simulink model "MKIV_build_simulink_flight_outer20210320_no1"  (R2016b)
settings: Solver=FixedStepDiscrete  StartTime=0.0  StopTime=inf  RelTol=1e-3
PostLoadFcn:
  | kFactor = 1.2;
  | 
  | KpRollAttitude = 0.630138625117681 / kFactor;
  | KiRollAttitude = 0.0552303199591522 / kFactor;
  | 
  | KpPitchAttitude = 0.630138625117681 / kFactor;
  | KiPitchAttitude = 0.0552303199591522 / kFactor;
  | 
  | KpRollRate = 1.31533836563383 / kFactor;
  | KiRollRate = 0.460338699849681 / kFactor;
  | 
  | KpPitchRate = 1.31533836563383 / kFactor;
  | KiPitchRate = 0.460338699849681 / kFactor;
  | 
  | KpYawRate = 1.31533836563383 / kFactor;
  | KiYawRate = 0.460338699849681 / kFactor;
undefined symbols (not defined in the file): PX4_TUNE_ENUM, RGBLED_COLOR_ENUM, RGBLED_MODE_ENUM
libraries: pixhawk_slib_sensors_actuators x8, pixhawk_slib_ADC_serial x1, pixhawk_slib_uORB_RW x1, pixhawk_slib_misc_utils x1
settings Model: Creator=Steve  LastModifiedBy=scott
settings SolverCC: AutoInsertRateTranBlk=on
settings DataIOCC: LimitDataPoints=on  SaveFormat=Array
settings OptimizationCC: DefaultParameterBehavior=Inlined  LifeSpan=1  MaxStackSize=64
settings DebuggingCC: SolverPrmCheckMsg=warning  AllowSymbolicDim=off  SFUnexpectedBacktrackingDiag=warning  SFNoUnconditionalDefaultTransitionDiag=warning  SFExecutionAtInitializationDiag=none
settings HardwareCC: ProdBitPerPointer=32  ProdBitPerSizeT=32  ProdBitPerPtrDiffT=32  ProdLargestAtomicInteger=Long  ProdLargestAtomicFloat=Double  ProdWordSize=32  ProdHWDeviceType=ARM Compatible->ARM Cortex
settings ModelReferenceCC: PropagateSignalLabelsOutOfModel=off
settings RTWCC: SystemTargetFile=ert.tlc  HardwareBoard=Pixhawk PX4  TemplateMakefile=ert_default_tmf  Description=Embedded Coder  GenerateReport=on  Toolchain=Pixhawk Toolchain  IncludeHyperlinkInReport=on  LaunchReport=on  GenerateTraceReport=on  GenerateTraceReportSl=on  GenerateTraceReportSf=on  GenerateTraceReportEml=on  GenerateCodeMetricsReport=on
settings CodeAppCC: IgnoreCustomStorageClasses=off
settings ERTTargetCC: CodeReplacementLibrary=GCC ARM Cortex-A9  ExtModeTransport=1  ExtModeMexFile=ext_serial_win32_comm  ExtModeMexArgs=/dev/serial  ERTCustomFileTemplate=PX4_codertarget_file_process.tlc  ConvertIfToSwitch=off  SuppressUnreachableDefaultCases=off
settings ConfigComp: CovMetricSettings=dw  CovHtmlReporting=on  CovSaveCumulativeToWorkspaceVar=on  CovSaveSingleToWorkspaceVar=on  CovExternalEMLEnable=off  CovSFcnEnable=off

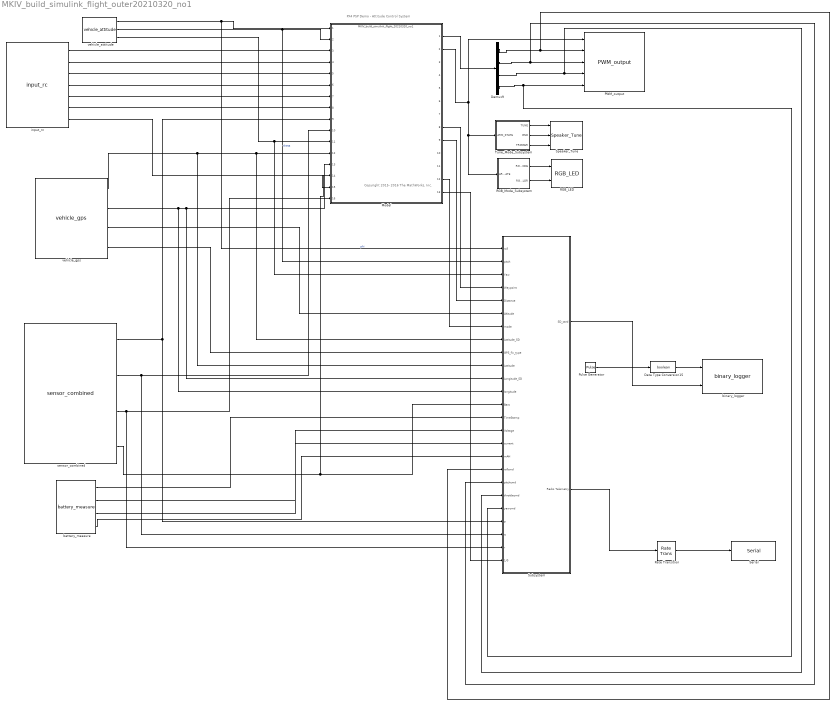
== system MKIV_build_simulink_flight_outer20210320_no1 ==
  note: PX4 PSP Demo - Attitude Control System
  note: Copyright 2015- 2016 The MathWorks, Inc.
  Data Type Conversion15 : DataTypeConversion  OutDataTypeStr=boolean
  Demux9 : Demux
  Model : ModelReference  ModelNameDialog=MKIV_build_simulink_flight_20210320_no1.slx  SimulationMode=Normal  ModelReferenceVersion=1.475
  PWM_output : pixhawk_slib_sensors_actuators/PWM_output  pwm_rate=50Hz  show_pwm1=on  show_pwm2=on  show_pwm3=on  show_pwm4=on  show_pwm5=off  show_pwm6=off  show_pwm7=off  show_pwm8=off
  Pulse Generator : DiscretePulseGenerator  Period=10  PulseWidth=5  SampleTime=10
  RGB_LED : pixhawk_slib_sensors_actuators/RGB_LED
  RGB_Mode_Subsystem : Subsystem
  Rate Transition : RateTransition  OutPortSampleTime=0.3
  Serial : pixhawk_slib_ADC_serial/Serial  DeviceName=/dev/ttyS1  ReadOrWrite=Writing  BaudRateStr=57600  block=on  WriteStatus=on  Terminator=off  Header=off  NumBytesRead=4  TerminatorChar=\n  HeaderData=57600  SimulateUsing=Code generation
  Speaker_Tune : pixhawk_slib_sensors_actuators/Speaker_Tune
  Subsystem : Subsystem
  Tune_Mode_Subsystem : Subsystem
  battery_measure : pixhawk_slib_sensors_actuators/battery_measure  SampleTime=1/250  VoltageOut=on  VoltageFilteredOut=off  CurrentOut=on  mAH_Out=on  TimeStamp=on
  binary_logger : pixhawk_slib_misc_utils/binary_logger  logfile=/fs/microsd/log  cacheflag=off  numRecs=1000
  input_rc : pixhawk_slib_sensors_actuators/input_rc  sampletime=1/250  channel1=on  channel2=on  channel3=on  channel4=on  channel5=on  channel6=on  channel7=on  channel8=off  ch_count=off  rssi=off  rc_failsafe=off  rc_lost=off  rc_inputsource=off
  sensor_combined : pixhawk_slib_sensors_actuators/sensor_combined  sampletime=1/250  show_mag=off  show_acc=off  show_gyro=on  show_baro=on  show_ts=off
  vehicle_attitude : pixhawk_slib_sensors_actuators/vehicle_attitude  sampletime=1/250  show_r=on  show_p=on  show_y=on  show_q=off
  vehicle_gps : pixhawk_slib_sensors_actuators/vehicle_gps  sampletime=1/250  show_ts_pos=off  show_alt=on  show_ts_gps=off  show_vel=off  show_fixtype=on  show_numsat=off
  wires:
  RGB_Mode_Subsystem/1(RGB_MODE) -> RGB_LED/1
  RGB_Mode_Subsystem/2(RGB_COLOR) -> RGB_LED/2
  Tune_Mode_Subsystem/1(TUNE) -> Speaker_Tune/1
  Tune_Mode_Subsystem/2(GND) -> Speaker_Tune/2
  Tune_Mode_Subsystem/3(TRIGGER) -> Speaker_Tune/3
  Model/2 -> RGB_Mode_Subsystem/1(ARM_STATE), Tune_Mode_Subsystem/1(ARM_STATE), PWM_output/1
  vehicle_attitude/2 -> Model/2, Subsystem/2(pitch)  "theta"
  input_rc/1 -> Model/3
  input_rc/2 -> Model/4
  input_rc/3 -> Model/5
  input_rc/4 -> Model/6
  input_rc/5 -> Model/7
  Model/1 -> Demux9/1
  input_rc/6 -> Model/8
  Rate Transition/1 -> Serial/1
  Subsystem/2(Radio Telemetry) -> Rate Transition/1
  vehicle_gps/1 -> Subsystem/8(Latitude_SD), Model/12, Subsystem/10(Latitude)
  vehicle_gps/2 -> Model/13, Subsystem/11(Longitude_SD), Subsystem/12(Iongitude)
  Data Type Conversion15/1 -> binary_logger/1
  Pulse Generator/1 -> Data Type Conversion15/1
  sensor_combined/4 -> Subsystem/13(Baro), Model/14
  input_rc/7 -> Model/15
  Model/8 -> Subsystem/4(Waypoint)
  Model/9 -> Subsystem/5(Distance)
  vehicle_gps/3 -> Subsystem/6(Altitude)
  Model/12 -> Subsystem/7(mode)
  vehicle_gps/4 -> Subsystem/9(GPS_fix_type)
  battery_measure/1 -> Subsystem/14(TimeStamp)
  battery_measure/2 -> Subsystem/15(Voltage)
  battery_measure/3 -> Subsystem/16("current ")
  battery_measure/4 -> Subsystem/17(mAH)
  Subsystem/1(SD_card) -> binary_logger/2
  Demux9/1 -> Subsystem/18(rollcmd), PWM_output/2
  Demux9/2 -> Subsystem/19(pitchcmd), PWM_output/3
  Demux9/3 -> Subsystem/20(throttlecmd), PWM_output/4
  Demux9/4 -> Subsystem/21(yawcmd), PWM_output/5
  sensor_combined/1 -> Model/9, Subsystem/22(p)
  sensor_combined/2 -> Subsystem/23(q), Model/10
  sensor_combined/3 -> Model/16, Subsystem/24(r)
  Model/13 -> Subsystem/25(1/0)
  vehicle_attitude/1 -> Subsystem/1(roll), Model/1  "phi"
  vehicle_attitude/3 -> Subsystem/3(Yaw), Model/11

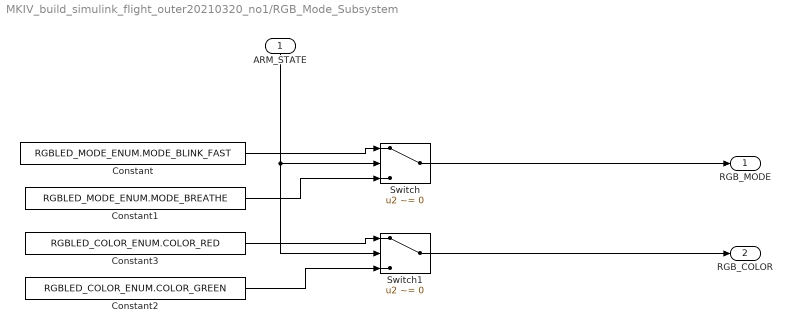
== system MKIV_build_simulink_flight_outer20210320_no1/RGB_Mode_Subsystem ==
  ARM_STATE : Inport
  Constant : Constant  Value=RGBLED_MODE_ENUM.MODE_BLINK_FAST  OutDataTypeStr=Enum: RGBLED_MODE_ENUM
  Constant1 : Constant  Value=RGBLED_MODE_ENUM.MODE_BREATHE  OutDataTypeStr=Enum: RGBLED_MODE_ENUM
  Constant2 : Constant  Value=RGBLED_COLOR_ENUM.COLOR_GREEN  OutDataTypeStr=Enum: RGBLED_COLOR_ENUM
  Constant3 : Constant  Value=RGBLED_COLOR_ENUM.COLOR_RED  OutDataTypeStr=Enum: RGBLED_COLOR_ENUM
  Switch : Switch  Criteria=u2 ~= 0  Threshold=1500  SampleTime=1/2
  Switch1 : Switch  Criteria=u2 ~= 0  Threshold=1500  SampleTime=1/2
  RGB_MODE : Outport
  RGB_COLOR : Outport  Port=2
  wires:
  ARM_STATE/1 -> Switch1/2, Switch/2
  Constant/1 -> Switch/1
  Constant1/1 -> Switch/3
  Switch/1 -> RGB_MODE/1
  Constant3/1 -> Switch1/1
  Constant2/1 -> Switch1/3
  Switch1/1 -> RGB_COLOR/1

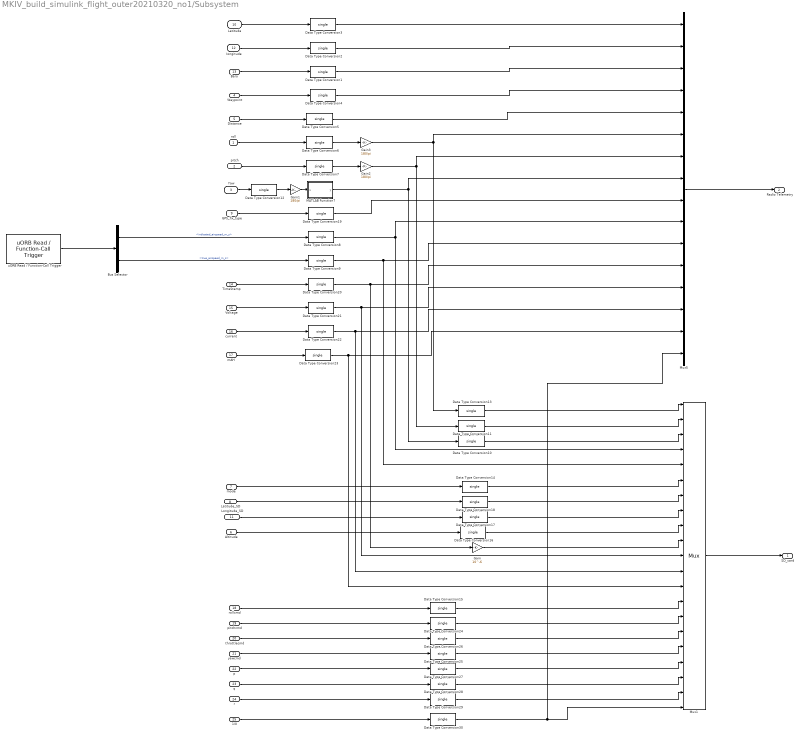
== system MKIV_build_simulink_flight_outer20210320_no1/Subsystem ==
  roll : Inport
  pitch : Inport  Port=2
  Yaw : Inport  Port=3
  Waypoint : Inport  Port=4
  Distance : Inport  Port=5
  Altitude : Inport  Port=6
  mode : Inport  Port=7
  Latitude_SD : Inport  Port=8
  GPS_fix_type : Inport  Port=9
  Latitude : Inport  Port=10
  Longitude_SD : Inport  Port=11
  Iongitude : Inport  Port=12
  Baro : Inport  Port=13
  TimeStamp : Inport  Port=14
  Voltage : Inport  Port=15
  "current " : Inport  Port=16
  mAH : Inport  Port=17
  rollcmd : Inport  Port=18
  pitchcmd : Inport  Port=19
  throttlecmd : Inport  Port=20
  yawcmd : Inport  Port=21
  p : Inport  Port=22
  q : Inport  Port=23
  r : Inport  Port=24
  1/0 : Inport  Port=25
  Bus Selector : BusSelector  OutputSignals=indicated_airspeed_m_s,true_airspeed_m_s
  Data Type Conversion{1..30} (30 alike) : DataTypeConversion  OutDataTypeStr=single
  Gain : Gain  Gain=10^-6
  Gain1 : Gain  Gain=180/pi
  Gain2 : Gain  Gain=180/pi
  Gain3 : Gain  Gain=180/pi
  MATLAB Function7 : MATLAB Function  TreatAsAtomicUnit=on
  Mux1 : Mux  Inputs=21
  Mux5 : Mux  Inputs=16
  uORB Read / Function-Call Trigger : pixhawk_slib_uORB_RW/uORB Read // Function-Call Trigger  uORB_Topic_str='airspeed'  BusObjVar=Bus: airspeed_SL  uORB_Interval=1  AsyncOutput=off  Fcn_call_select=Generate Function Call Signal  TaskName='Task1'  Poll_timeout=100  Ts=-1
  SD_card : Outport
  Radio Telemetry : Outport  Port=2
  wires:
  Data Type Conversion4/1 -> Mux5/4
  Gain3/1 -> Data Type Conversion13/1, Mux5/6
  Data Type Conversion3/1 -> Mux5/1
  Data Type Conversion2/1 -> Mux5/2
  Gain1/1 -> MATLAB Function7/1(u)
  Data Type Conversion11/1 -> Mux1/2
  Data Type Conversion7/1 -> Gain2/1
  Mux1/1 -> SD_card/1
  Gain2/1 -> Data Type Conversion11/1, Mux5/7
  Waypoint/1 -> Data Type Conversion4/1
  Data Type Conversion14/1 -> Mux1/6
  Data Type Conversion13/1 -> Mux1/1
  Data Type Conversion1/1 -> Mux5/3
  Data Type Conversion6/1 -> Gain3/1
  Data Type Conversion5/1 -> Mux5/5
  Data Type Conversion8/1 -> Mux5/10, Mux1/4
  Data Type Conversion9/1 -> Mux5/11, Mux1/5
  Data Type Conversion12/1 -> Gain1/1
  mode/1 -> Data Type Conversion14/1
  Data Type Conversion10/1 -> Mux1/3
  Distance/1 -> Data Type Conversion5/1
  MATLAB Function7/1(y) -> Data Type Conversion10/1, Mux5/8
  mAH/1 -> Data Type Conversion23/1
  Data Type Conversion21/1 -> Mux5/13, Mux1/11
  GPS_fix_type/1 -> Data Type Conversion19/1
  "current "/1 -> Data Type Conversion22/1
  Altitude/1 -> Data Type Conversion16/1
  Bus Selector/1 -> Data Type Conversion8/1  "<indicated_airspeed_m_s>"
  Data Type Conversion19/1 -> Mux5/9
  Data Type Conversion23/1 -> Mux5/15, Mux1/13
  Voltage/1 -> Data Type Conversion21/1
  Data Type Conversion17/1 -> Mux1/8
  Data Type Conversion18/1 -> Mux1/7
  uORB Read / Function-Call Trigger/1 -> Bus Selector/1
  TimeStamp/1 -> Data Type Conversion20/1
  Data Type Conversion20/1 -> Mux5/12, Gain/1
  Data Type Conversion22/1 -> Mux5/14, Mux1/12
  Gain/1 -> Mux1/10
  Bus Selector/2 -> Data Type Conversion9/1  "<true_airspeed_m_s>"
  Data Type Conversion16/1 -> Mux1/9
  Baro/1 -> Data Type Conversion1/1
  Iongitude/1 -> Data Type Conversion2/1
  Latitude/1 -> Data Type Conversion3/1
  Latitude_SD/1 -> Data Type Conversion18/1
  Longitude_SD/1 -> Data Type Conversion17/1
  pitch/1 -> Data Type Conversion7/1
  Yaw/1 -> Data Type Conversion12/1
  roll/1 -> Data Type Conversion6/1
  Mux5/1 -> Radio Telemetry/1
  rollcmd/1 -> Data Type Conversion15/1
  pitchcmd/1 -> Data Type Conversion24/1
  throttlecmd/1 -> Data Type Conversion26/1
  yawcmd/1 -> Data Type Conversion25/1
  Data Type Conversion15/1 -> Mux1/14
  Data Type Conversion24/1 -> Mux1/15
  Data Type Conversion26/1 -> Mux1/16
  Data Type Conversion25/1 -> Mux1/17
  Data Type Conversion27/1 -> Mux1/18
  Data Type Conversion28/1 -> Mux1/19
  Data Type Conversion29/1 -> Mux1/20
  p/1 -> Data Type Conversion27/1
  q/1 -> Data Type Conversion28/1
  r/1 -> Data Type Conversion29/1
  1/0/1 -> Data Type Conversion30/1
  Data Type Conversion30/1 -> Mux5/16, Mux1/21

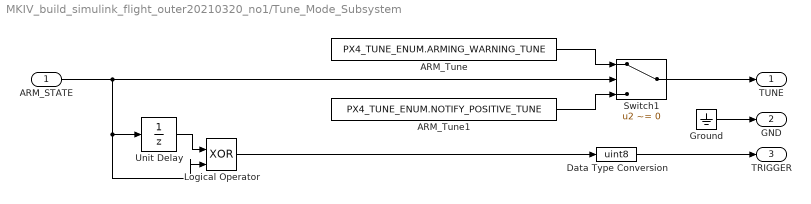
== system MKIV_build_simulink_flight_outer20210320_no1/Tune_Mode_Subsystem ==
  ARM_STATE : Inport
  ARM_Tune : Constant  Value=PX4_TUNE_ENUM.ARMING_WARNING_TUNE  OutDataTypeStr=Enum: PX4_TUNE_ENUM
  ARM_Tune1 : Constant  Value=PX4_TUNE_ENUM.NOTIFY_POSITIVE_TUNE  OutDataTypeStr=Enum: PX4_TUNE_ENUM
  Data Type Conversion : DataTypeConversion  OutDataTypeStr=uint8
  Ground : Ground
  Logical Operator : Logic  Operator=XOR  IconShape=distinctive  AllPortsSameDT=off  OutDataTypeStr=boolean
  Switch1 : Switch  Criteria=u2 ~= 0  Threshold=1500
  Unit Delay : UnitDelay  SampleTime=-1
  TUNE : Outport
  GND : Outport  Port=2
  TRIGGER : Outport  Port=3
  wires:
  Ground/1 -> GND/1
  Data Type Conversion/1 -> TRIGGER/1
  Switch1/1 -> TUNE/1
  ARM_Tune/1 -> Switch1/1
  ARM_Tune1/1 -> Switch1/3
  ARM_STATE/1 -> Logical Operator/2, Unit Delay/1, Switch1/2
  Unit Delay/1 -> Logical Operator/1
  Logical Operator/1 -> Data Type Conversion/1

== matlab function MKIV_build_simulink_flight_outer20210320_no1/Subsystem/MATLAB Function7 ==
  data: u input; y output
function y = fcn(u)
if(u<=0)
    y=360+u;
else
    y=u
end
